simulink library "TurbochargingEngLib"  (R2013a)
settings: Solver=ode45  StartTime=0.0  StopTime=10.0  FixedStep=1e-4  RelTol=1e-3
undefined symbols (not defined in the file): comp_eff_map, comp_flow_map, D_turb_wheel, eff_coeff, eta_turb_max, flow_coeff_turb, fs, J_tc, jTC, n288_rep, npr, nsp, omegat0, pr_rep, RPMT0, T_ref_turb, Uc_opt
libraries: EngineSysteSubmodel x4
settings Model: Creator=yum  LastModifiedBy=yum

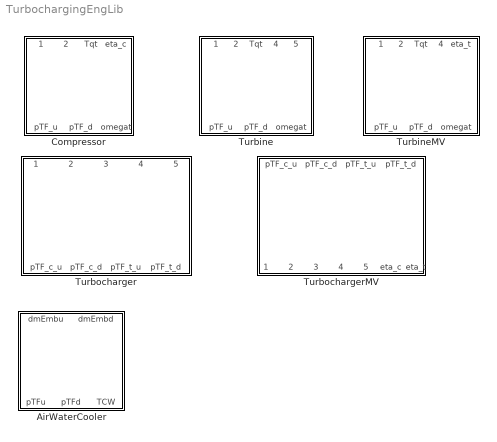
== system TurbochargingEngLib ==
  AirWaterCooler : Subsystem  mask{fs=0, Cd=0, A_air_path=0, dm_cw=0, coeff_T_cw_K=0, Cp_cw=0, D_cw_pipe=0}
      mask prompts: fs "Stoichiometric fuel-air ratio"; Cd "Discharge coefficient (0.8)"; A_air_path "Effective sectional area of air path (m2)"; dm_cw "Coolant flow rate (kg/s)"; coeff_T_cw_K "Coefficient for effective heat transfer area w.r.t. coolant temperature (2x1)"; Cp_cw "Specific heat capacity of coolant"; D_cw_pipe "Pipe diameter of the cooling water pipe in the cooler (m)"
      mask TypeOptions fs: S-Function/fs
      mask TypeOptions Cd: S-Function/Cd
      mask TypeOptions A_air_path: S-Function/A_air_path
      mask TypeOptions dm_cw: S-Function/dm_cw
      mask TypeOptions coeff_T_cw_K: S-Function/coeff_T_cw_K
      mask TypeOptions Cp_cw: S-Function/Cp_cw
      mask TypeOptions D_cw_pipe: S-Function/D_cw_pipe
  Compressor : Subsystem  mask{fs=0, comp_flow_map=0, comp_eff_map=0, pr_rep=0, n288_rep=0, npr=0, nsp=0}
      mask prompts: fs "Fuel-air equivalent ratio"; comp_flow_map "Compressor map for corrected flow"; comp_eff_map "Compressor map for efficiency"; pr_rep "Pressure ratio array for look-up in compressor map"; n288_rep "Corrected speed array for look-up in compressor map"; npr "Length of pressure ratio array for look-up in compressor map"; nsp "Length of corrected speed array for look-up in compressor map"
  Turbine : Subsystem  mask{fs=0, flow_coeff_turb=0, eff_coeff=0}
      mask prompts: fs "Fuel-Air equivalent ratio"; flow_coeff_turb "Turbine flow coefficient"; eff_coeff "Turbine efficient coefficient"
      mask TypeOptions fs: S-Function/fs
      mask TypeOptions flow_coeff_turb: S-Function/flow_coeff_turb
      mask TypeOptions eff_coeff: S-Function/eff_coeff
  TurbineMV : Subsystem  AncestorBlock=EngineSysteSubmodel/TurbineMV  mask{fs=0, flow_coeff_turb=0, D_turb_wheel=0, Uc_opt=0, eta_turb_max=0}
      mask prompts: fs "Stoichiometric fuel-air ratio"; flow_coeff_turb "Flow coefficient for turbine model (3x1)"; D_turb_wheel "Turbine wheel diameter (m)"; Uc_opt "Optimal blade speed ratio"; eta_turb_max "Maximum efficiency"
  Turbocharger : Subsystem  mask{fs=fs, jTC=jTC, comp_flow_map=comp_flow_map, comp_eff_map=comp_eff_map, pr_rep=pr_rep, n288_rep=n288_rep, npr=npr, nsp=nsp, flow_coeff_turb=flow_coeff_turb, eff_coeff=eff_coeff, omegat0=RPMT0 * pi / 30}
      mask prompts: fs "Stoichiometric fuel-air ratio"; jTC "Mass moment of inertia of a rotor (kgm2)"; comp_flow_map "Compressor map for corrected flow"; comp_eff_map "Compressor map for efficiency"; pr_rep "Pressure ratio array for look-up in compressor map"; n288_rep "Corrected speed array for look-up in compressor map"; npr "Length of pressure ratio array for look-up in compressor map"; nsp "Length of corrected speed array for look-up in compressor map"; flow_coeff_turb "Turbine flow coefficient"; eff_coeff "Turbine efficient coefficient"; omegat0 "Initial rotating speed (rad/s)"
      mask TypeOptions fs: Compressor1/fs | Turbine1/fs
      mask TypeOptions comp_flow_map: Compressor1/comp_flow_map
      mask TypeOptions comp_eff_map: Compressor1/comp_eff_map
      mask TypeOptions pr_rep: Compressor1/pr_rep
      mask TypeOptions n288_rep: Compressor1/n288_rep
      mask TypeOptions npr: Compressor1/npr
      mask TypeOptions nsp: Compressor1/nsp
      mask TypeOptions flow_coeff_turb: Turbine1/flow_coeff_turb
      mask TypeOptions eff_coeff: Turbine1/eff_coeff
  TurbochargerMV : Subsystem  mask{fs=fs, J_tc=J_tc, omegat0=omegat0, comp_flow_map=comp_flow_map, comp_eff_map=comp_eff_map, pr_rep=pr_rep, n_288_rep=n288_rep, npr=npr, nsp=nsp, flow_coeff_turb=flow_coeff_turb, D_wheel_turb=D_turb_wheel, Uc_opt=Uc_opt, eta_turb_max=eta_turb_max, T_ref=T_ref_turb}
      mask prompts: fs "Stoichiometric fuel-air ratio"; J_tc "Mass moment of inertia of a rotor"; omegat0 "Initial rotor speed"; comp_flow_map "Compressor map for corrected flow"; comp_eff_map "Compressor map for efficiency"; pr_rep "Pressure ratio arry for look-up in compressor map"; n_288_rep "Corrected speed array for look-up in compressor map"; npr "Length of pressure ratio array for look-up in compressor map"; nsp "Length of corrected speed array for look-up in compressor map"; flow_coeff_turb "Flow coefficient for turbine model"; D_wheel_turb "Turbine wheel diameter"; Uc_opt "Optimal blade speed ratio"; eta_turb_max "Maximum efficiency"; T_ref "Reference temperature for turbine flow"

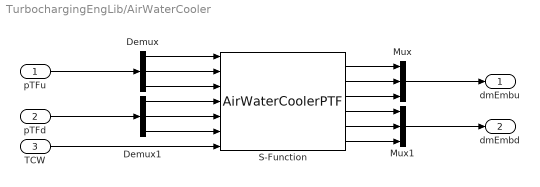
== system TurbochargingEngLib/AirWaterCooler ==
  pTFu : Inport
  pTFd : Inport  Port=2
  TCW : Inport  Port=3
  Demux : Demux  Outputs=3
  Demux1 : Demux  Outputs=3
  Mux : Mux  Inputs=3
  Mux1 : Mux  Inputs=3
  S-Function : S-Function  FunctionName=AirWaterCoolerPTF  Parameters=fs,Cd,A_air_path,dm_cw,coeff_T_cw_K,Cp_cw,D_cw_pipe  SFunctionModules='GetAirDensity GetAirThermalConduct GetAirViscosity GetCompCombGas_rtwutil GetHTCoeffHTX GetIdealNozzleFlow GetThdynCombGasZach rt_nonfinite rtGetInf rtGetNaN'  EnableBusSupport=off  mask{fs=fs, Cd=Cd, A_air_path=A_air_path, dm_cw=dm_cw, coeff_T_cw_K=coeff_T_cw_K, Cp_cw=Cp_cw, D_cw_pipe=D_cw_pipe}
      mask prompts: fs "Stoichiometric fuel-air ratio"; Cd "Discharge coefficient (0.8)"; A_air_path "Effective sectional area of air path (m2)"; dm_cw "Coolant flow rate (kg/s)"; coeff_T_cw_K "Coefficient for effective heat transfer area w.r.t. coolant temperature (2x1)"; Cp_cw "Specific heat capacity of coolant"; D_cw_pipe "Pipe diameter of the cooling water pipe in the cooler (m)"
  dmEmbu : Outport
  dmEmbd : Outport  Port=2
  wires:
  S-Function/6 -> Mux1/3
  S-Function/5 -> Mux1/2
  S-Function/4 -> Mux1/1
  S-Function/3 -> Mux/3
  S-Function/2 -> Mux/2
  S-Function/1 -> Mux/1
  Demux/1 -> S-Function/1
  Demux/3 -> S-Function/3
  Demux/2 -> S-Function/2
  Demux1/3 -> S-Function/6
  Demux1/1 -> S-Function/4
  Demux1/2 -> S-Function/5
  pTFd/1 -> Demux1/1
  pTFu/1 -> Demux/1
  Mux/1 -> dmEmbu/1
  Mux1/1 -> dmEmbd/1
  TCW/1 -> S-Function/7

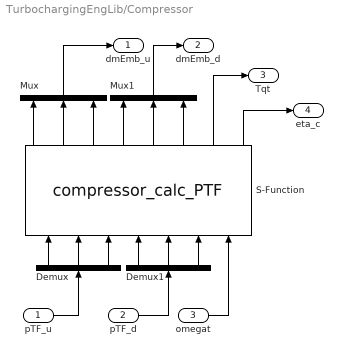
== system TurbochargingEngLib/Compressor ==
  pTF_u : Inport
  pTF_d : Inport  Port=2
  omegat : Inport  Port=3
  Demux : Demux  Outputs=3
  Demux1 : Demux  Outputs=3
  Mux : Mux  Inputs=3
  Mux1 : Mux  Inputs=3
  S-Function : S-Function  FunctionName=compressor_calc_PTF  Parameters=fs,comp_flow_map,comp_eff_map,pr_rep,n288_rep,int32(npr),int32(nsp)  SFunctionModules=GetThdynCombGasZach.c  EnableBusSupport=off
  dmEmb_u : Outport
  dmEmb_d : Outport  Port=2
  Tqt : Outport  Port=3
  eta_c : Outport  Port=4
  wires:
  Demux/1 -> S-Function/1
  Demux/3 -> S-Function/3
  Demux/2 -> S-Function/2
  Demux1/2 -> S-Function/5
  Demux1/3 -> S-Function/6
  Demux1/1 -> S-Function/4
  pTF_d/1 -> Demux1/1
  omegat/1 -> S-Function/7
  pTF_u/1 -> Demux/1
  S-Function/5 -> Mux1/2
  S-Function/4 -> Mux1/1
  S-Function/6 -> Mux1/3
  S-Function/1 -> Mux/1
  S-Function/2 -> Mux/2
  S-Function/3 -> Mux/3
  Mux/1 -> dmEmb_u/1
  Mux1/1 -> dmEmb_d/1
  S-Function/7 -> Tqt/1
  S-Function/8 -> eta_c/1

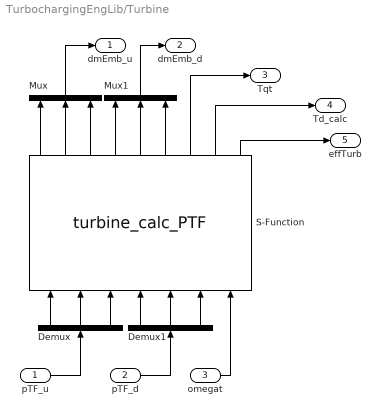
== system TurbochargingEngLib/Turbine ==
  pTF_u : Inport
  pTF_d : Inport  Port=2
  omegat : Inport  Port=3
  Demux : Demux  Outputs=3
  Demux1 : Demux  Outputs=3
  Mux : Mux  Inputs=3
  Mux1 : Mux  Inputs=3
  S-Function : S-Function  FunctionName=turbine_calc_PTF  Parameters=fs,flow_coeff_turb,eff_coeff  SFunctionModules=GetThdynCombGasZach.c  EnableBusSupport=off  mask{fs=fs, flow_coeff_turb=flow_coeff_turb, eff_coeff=eff_coeff}
      mask prompts: fs "Stoichiometric fuel air ratio"; flow_coeff_turb "Coefficient for flow model of turbine"; eff_coeff "Coefficient for efficiency model of turbine"
  dmEmb_u : Outport
  dmEmb_d : Outport  Port=2
  Tqt : Outport  Port=3
  Td_calc : Outport  Port=4
  effTurb : Outport  Port=5
  wires:
  Demux/1 -> S-Function/1
  Demux/3 -> S-Function/3
  Demux/2 -> S-Function/2
  Demux1/2 -> S-Function/5
  Demux1/3 -> S-Function/6
  Demux1/1 -> S-Function/4
  pTF_d/1 -> Demux1/1
  omegat/1 -> S-Function/7
  pTF_u/1 -> Demux/1
  S-Function/8 -> Td_calc/1
  S-Function/5 -> Mux1/2
  S-Function/4 -> Mux1/1
  S-Function/6 -> Mux1/3
  S-Function/1 -> Mux/1
  S-Function/2 -> Mux/2
  S-Function/3 -> Mux/3
  Mux/1 -> dmEmb_u/1
  Mux1/1 -> dmEmb_d/1
  S-Function/7 -> Tqt/1
  S-Function/9 -> effTurb/1

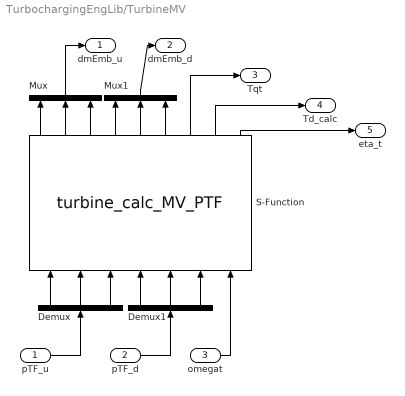
== system TurbochargingEngLib/TurbineMV ==
  pTF_u : Inport
  pTF_d : Inport  Port=2
  omegat : Inport  Port=3
  Demux : Demux  Outputs=3
  Demux1 : Demux  Outputs=3
  Mux : Mux  Inputs=3
  Mux1 : Mux  Inputs=3
  S-Function : S-Function  FunctionName=turbine_calc_MV_PTF  Parameters=fs,flow_coeff_turb,D_turb_wheel,Uc_opt,eta_turb_max,T_ref_turb  SFunctionModules=GetThdynCombGasZach.c  EnableBusSupport=off
  dmEmb_u : Outport
  dmEmb_d : Outport  Port=2
  Tqt : Outport  Port=3
  Td_calc : Outport  Port=4
  eta_t : Outport  Port=5
  wires:
  Demux/1 -> S-Function/1
  Demux/3 -> S-Function/3
  Demux/2 -> S-Function/2
  Demux1/2 -> S-Function/5
  Demux1/3 -> S-Function/6
  Demux1/1 -> S-Function/4
  pTF_d/1 -> Demux1/1
  omegat/1 -> S-Function/7
  pTF_u/1 -> Demux/1
  S-Function/8 -> Td_calc/1
  S-Function/5 -> Mux1/2
  S-Function/4 -> Mux1/1
  S-Function/6 -> Mux1/3
  S-Function/1 -> Mux/1
  S-Function/2 -> Mux/2
  S-Function/3 -> Mux/3
  Mux/1 -> dmEmb_u/1
  Mux1/1 -> dmEmb_d/1
  S-Function/7 -> Tqt/1
  S-Function/9 -> eta_t/1

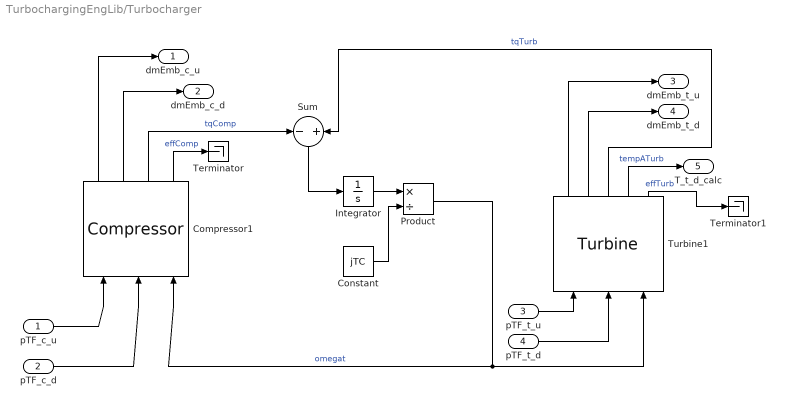
== system TurbochargingEngLib/Turbocharger ==
  pTF_c_u : Inport
  pTF_c_d : Inport  Port=2
  pTF_t_u : Inport  Port=3
  pTF_t_d : Inport  Port=4
  Compressor1 : EngineSysteSubmodel/Compressor  fs=fs  comp_flow_map=comp_flow_map  comp_eff_map=comp_eff_map  pr_rep=pr_rep  n288_rep=n288_rep  npr=npr  nsp=nsp
  Constant : Constant  Value=jTC
  Integrator : Integrator  InitialCondition=omegat0*jTC
  Product : Product  Inputs=*/
  Sum : Sum  Inputs=-|+
  Terminator : Terminator
  Terminator1 : Terminator
  Turbine1 : EngineSysteSubmodel/Turbine  fs=fs  flow_coeff_turb=flow_coeff_turb  eff_coeff=eff_coeff
  dmEmb_c_u : Outport
  dmEmb_c_d : Outport  Port=2
  dmEmb_t_u : Outport  Port=3
  dmEmb_t_d : Outport  Port=4
  T_t_d_calc : Outport  Port=5
  wires:
  pTF_c_d/1 -> Compressor1/2
  Turbine1/3 -> Sum/2  "tqTurb"
  Turbine1/1 -> dmEmb_t_u/1
  Compressor1/1 -> dmEmb_c_u/1
  Product/1 -> Turbine1/3, Compressor1/3  "omegat"
  Compressor1/2 -> dmEmb_c_d/1
  Integrator/1 -> Product/1
  Sum/1 -> Integrator/1
  Compressor1/3 -> Sum/1  "tqComp"
  Turbine1/2 -> dmEmb_t_d/1
  Turbine1/4 -> T_t_d_calc/1  "tempATurb"
  pTF_c_u/1 -> Compressor1/1
  pTF_t_u/1 -> Turbine1/1
  pTF_t_d/1 -> Turbine1/2
  Constant/1 -> Product/2
  Compressor1/4 -> Terminator/1  "effComp"
  Turbine1/5 -> Terminator1/1  "effTurb"

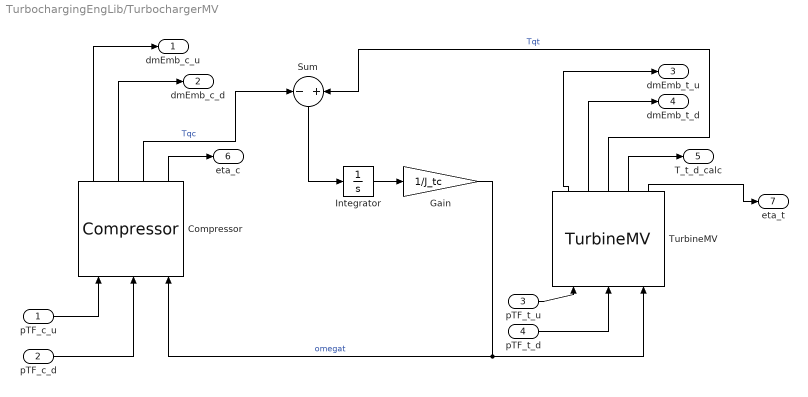
== system TurbochargingEngLib/TurbochargerMV ==
  pTF_c_u : Inport
  pTF_c_d : Inport  Port=2
  pTF_t_u : Inport  Port=3
  pTF_t_d : Inport  Port=4
  Compressor : EngineSysteSubmodel/Compressor  fs=fs  comp_flow_map=comp_flow_map  comp_eff_map=comp_eff_map  pr_rep=pr_rep  n288_rep=n288_rep  npr=npr  nsp=nsp
  Gain : Gain  Gain=1/J_tc
  Integrator : Integrator  InitialCondition=omegat0*J_tc
  Sum : Sum  Inputs=-|+
  TurbineMV : EngineSysteSubmodel/TurbineMV  fs=fs  flow_coeff_turb=flow_coeff_turb  D_turb_wheel=D_turb_wheel  Uc_opt=Uc_opt  eta_turb_max=eta_turb_max
  dmEmb_c_u : Outport
  dmEmb_c_d : Outport  Port=2
  dmEmb_t_u : Outport  Port=3
  dmEmb_t_d : Outport  Port=4
  T_t_d_calc : Outport  Port=5
  eta_c : Outport  Port=6
  eta_t : Outport  Port=7
  wires:
  TurbineMV/5 -> eta_t/1
  TurbineMV/3 -> Sum/2  "Tqt"
  TurbineMV/1 -> dmEmb_t_u/1
  Compressor/1 -> dmEmb_c_u/1
  Gain/1 -> Compressor/3, TurbineMV/3  "omegat"
  Compressor/2 -> dmEmb_c_d/1
  Integrator/1 -> Gain/1
  Sum/1 -> Integrator/1
  Compressor/3 -> Sum/1  "Tqc"
  TurbineMV/2 -> dmEmb_t_d/1
  TurbineMV/4 -> T_t_d_calc/1
  pTF_c_d/1 -> Compressor/2
  pTF_c_u/1 -> Compressor/1
  pTF_t_u/1 -> TurbineMV/1
  pTF_t_d/1 -> TurbineMV/2
  Compressor/4 -> eta_c/1
